simulink model "Prueba2"  (R2017b)
settings: Solver=FixedStepAuto  StartTime=0.0  StopTime=10.0  RelTol=1e-3  EnableMultiTasking=on
undefined symbols (not defined in the file): Color, encod_L, encod_R, Gyro, Ultra
libraries: legoev3lib x12
settings Model: ExtModeTrigDuration=2  Creator=Nexel  LastModifiedBy=Nexel
settings SolverCC: PositivePriorityOrder=on
settings OptimizationCC: PassReuseOutputArgsThreshold=0  MaxStackSize=64
settings DebuggingCC: ParameterTunabilityLossMsg=error
settings HardwareCC: ProdBitPerPointer=32  ProdBitPerSizeT=32  ProdBitPerPtrDiffT=32  ProdLargestAtomicInteger=Long  ProdWordSize=32  ProdHWDeviceType=ARM Compatible->ARM 9  UseEmbeddedCoderFeatures=off  UseSimulinkCoderFeatures=off
settings SFSimCC: MATLABDynamicMemAlloc=off
settings RTWCC: SystemTargetFile=ert.tlc  HardwareBoard=LEGO MINDSTORMS EV3  TemplateMakefile=ert_default_tmf  GenerateReport=on  Toolchain=Sourcery G++ Lite v2009q3  LaunchReport=on
settings CodeAppCC: ForceParamTrailComments=on  OperatorAnnotations=on
settings ERTTargetCC: ERTCustomFileBanners=off  SupportContinuousTime=on  SupportNonInlinedSFcns=on  RemoveResetFunc=off  SupportVariableSizeSignals=on  ModelStepFunctionPrototypeControlCompliant=off

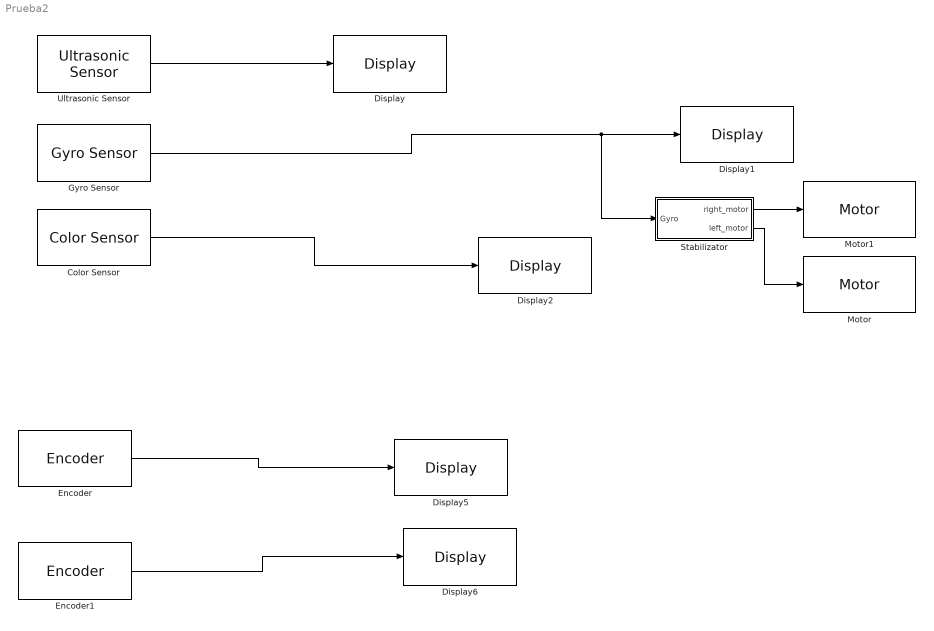
== system Prueba2 ==
  Color Sensor : legoev3lib/Color Sensor  portNumber=3  mode=Reflected light intensity  sampleTime=0.1
      settings: SourceProductName=Simulink Support Package for LEGO MINDSTORMS EV3 Hardware  SourceProductBaseCode=LEGOEV3
  Display : legoev3lib/Display  slcdStr=Ultra:  slcdLine=2  slcdFormat=Decimal
      settings: SourceProductName=Simulink Support Package for LEGO MINDSTORMS EV3 Hardware  SourceProductBaseCode=LEGOEV3
  Display1 : legoev3lib/Display  slcdStr=Gyro:  slcdLine=3  slcdFormat=Decimal
      settings: SourceProductName=Simulink Support Package for LEGO MINDSTORMS EV3 Hardware  SourceProductBaseCode=LEGOEV3
  Display2 : legoev3lib/Display  slcdStr=Color:  slcdLine=4  slcdFormat=Decimal
      settings: SourceProductName=Simulink Support Package for LEGO MINDSTORMS EV3 Hardware  SourceProductBaseCode=LEGOEV3
  Display5 : legoev3lib/Display  slcdStr=encod_L:  slcdLine=7  slcdFormat=Decimal
      settings: SourceProductName=Simulink Support Package for LEGO MINDSTORMS EV3 Hardware  SourceProductBaseCode=LEGOEV3
  Display6 : legoev3lib/Display  slcdStr=encod_R:  slcdLine=8  slcdFormat=Decimal
      settings: SourceProductName=Simulink Support Package for LEGO MINDSTORMS EV3 Hardware  SourceProductBaseCode=LEGOEV3
  Encoder : legoev3lib/Encoder  portNumber=C  opMode=No reset  sampleTime=0.1
      settings: SourceProductName=Simulink Support Package for LEGO MINDSTORMS EV3 Hardware  SourceProductBaseCode=LEGOEV3
  Encoder1 : legoev3lib/Encoder  portNumber=B  opMode=No reset  sampleTime=0.1
      settings: SourceProductName=Simulink Support Package for LEGO MINDSTORMS EV3 Hardware  SourceProductBaseCode=LEGOEV3
  Gyro Sensor : legoev3lib/Gyro Sensor  portNumber=2  sampleTime=0.1
      settings: SourceProductName=Simulink Support Package for LEGO MINDSTORMS EV3 Hardware  SourceProductBaseCode=LEGOEV3
  Motor : legoev3lib/Motor  sportNumber=C  sstopAction=Brake
  Motor1 : legoev3lib/Motor  sportNumber=B  sstopAction=Brake
  Stabilizator : Subsystem
  Ultrasonic Sensor : legoev3lib/Ultrasonic Sensor  PortNumber=4  sampleTime=0.1
      settings: SourceProductName=Simulink Support Package for LEGO MINDSTORMS EV3 Hardware  SourceProductBaseCode=LEGOEV3
  wires:
  Encoder/1 -> Display5/1
  Encoder1/1 -> Display6/1
  Gyro Sensor/1 -> Stabilizator/1("Gyro "), Display1/1
  Ultrasonic Sensor/1 -> Display/1
  Stabilizator/2("left_motor ") -> Motor/1
  Stabilizator/1("right_motor ") -> Motor1/1
  Color Sensor/1 -> Display2/1

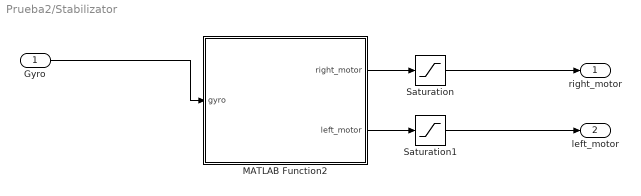
== system Prueba2/Stabilizator ==
  "Gyro " : Inport
  MATLAB Function2 : MATLAB Function  TreatAsAtomicUnit=on
  Saturation : Saturate  UpperLimit=+80  LowerLimit=-80
  Saturation1 : Saturate  UpperLimit=+80  LowerLimit=-80
  "right_motor " : Outport
  "left_motor " : Outport  Port=2
  wires:
  "Gyro "/1 -> MATLAB Function2/1(gyro)
  Saturation/1 -> "right_motor "/1
  Saturation1/1 -> "left_motor "/1
  MATLAB Function2/1(right_motor) -> Saturation/1
  MATLAB Function2/2(left_motor) -> Saturation1/1

== matlab function Prueba2/Stabilizator/MATLAB Function2 ==
  data: right_motor output; gyro input; left_motor output
function [right_motor, left_motor] = stabilizator(gyro)
    persistent last_right_motor
    persistent last_left_motor
    if isempty(last_right_motor)
        last_right_motor = 0;
        last_left_motor = 0;
    end
    added_power = 5;
    if gyro < 50
        left_motor = last_left_motor - added_power;
        right_motor = last_right_motor - added_power;
    elseif gyro > 50
        left_motor = last_left_motor + added_power;
        right_motor = last_right_motor + added_power;
    else
        left_motor = last_left_motor;
        right_motor = last_right_motor;
    end
        last_right_motor = right_motor;
        last_left_motor = left_motor;
end
